simulink model "H250_LOEUnknown_400HzV3"  (R2022a)
settings: Solver=ode4  StartTime=0.0  StopTime=80  FixedStep=Ts  RelTol=1e-3
InitFcn:
  | H250_LOEUnknown_400HzParam
undefined symbols (not defined in the file or in its folder): DiscIntNeverNeededParam, Ts
libraries: sharedtransform x3, dspnetwork x1, pixhawk_slib_misc_utils x1
settings Model: Creator=kcx06  LastModifiedBy=kcx06
settings SolverCC: AlgebraicLoopSolver=TrustRegion  PositivePriorityOrder=on  AutoInsertRateTranBlk=on
settings DataIOCC: SaveOutput=off  DSMLogging=off  SaveTime=off  ReturnWorkspaceOutputs=off
settings OptimizationCC: DefaultParameterBehavior=Inlined  EnhancedBackFolding=on  PassReuseOutputArgsAs=Individual arguments  ZeroExternalMemoryAtStartup=off  ZeroInternalMemoryAtStartup=off  MaxStackSize=64  OptimizeBlockOrder=speed  DifferentSizesBufferReuse=on  OptimizationCustomize=off  EfficientTunableParamExpr=on
settings DebuggingCC: ParameterTunabilityLossMsg=error  UnconnectedInputMsg=warning  UnconnectedOutputMsg=warning  UnconnectedLineMsg=warning  SFMachineParentedDataDiag=warning
settings HardwareCC: ProdBitPerPointer=32  ProdBitPerSizeT=32  ProdBitPerPtrDiffT=32  ProdLargestAtomicInteger=Long  ProdLargestAtomicFloat=Double  ProdWordSize=32  ProdHWDeviceType=ARM Compatible->ARM Cortex
settings SFSimCC: MATLABDynamicMemAlloc=off
settings RTWCC: SystemTargetFile=ert.tlc  HardwareBoard=Pixhawk PX4  TLCOptions="-aInlineSetEventsForThisBaseRateFcn=TLC_FALSE -aSuppressMultiTaskScheduler=TLC_FALSE  -aRateBasedStepFcn=0"  TemplateMakefile=ert_default_tmf  GenerateReport=on  CustomSource=px4_simulink_app_params.c  Toolchain=Pixhawk Toolchain  BuildConfiguration=Faster Runs  LaunchReport=on  DLArmComputeVersion=19.05
settings CodeAppCC: ForceParamTrailComments=on  IgnoreCustomStorageClasses=off  OperatorAnnotations=on  SimulinkDataObjDesc=on  SFDataObjDesc=on  InsertBlockDesc=on
settings ERTTargetCC: SupportComplex=off  SupportContinuousTime=on  InlinedParameterPlacement=NonHierarchical  ERTCustomFileTemplate=px4_codertarget_file_process.tlc

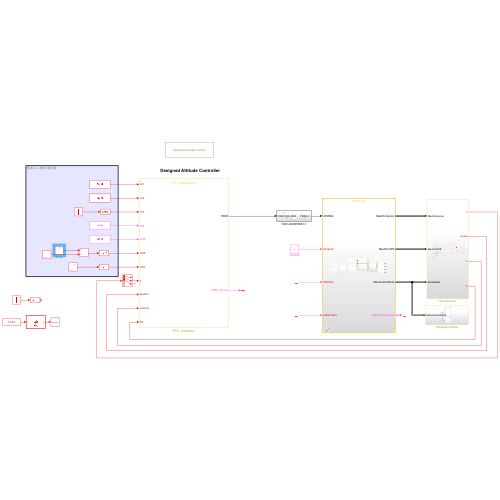
[thumbnail: Simulink's stored preview of the top-level diagram]
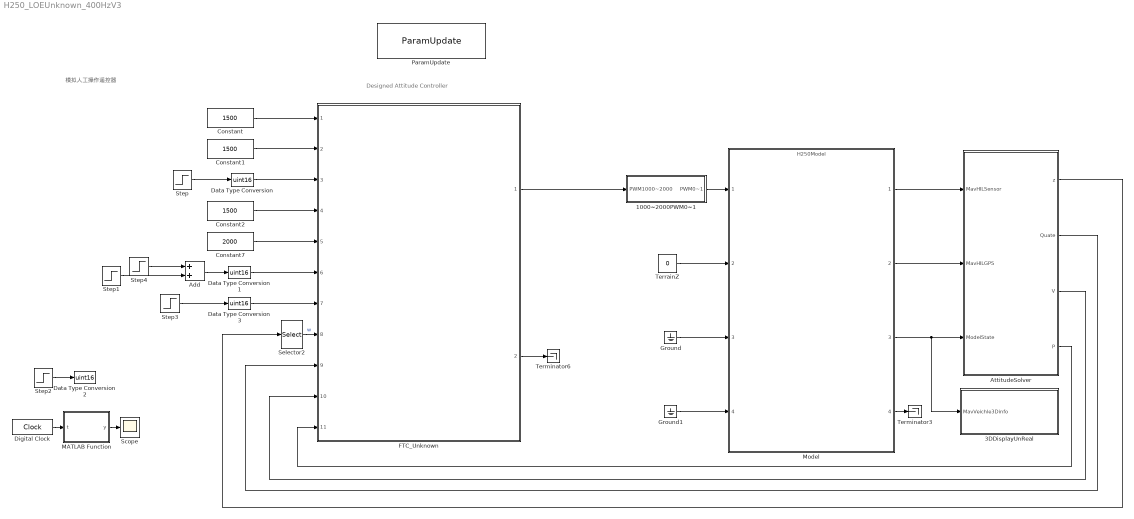
== system H250_LOEUnknown_400HzV3 ==
  note: Designed Attitude Controller
  note: 模拟人工操作遥控器
  1000~2000PWM0~1 : Subsystem
  3DDisplayUnReal : Subsystem
  Add : Sum
  AttitudeSolver : Subsystem
  Constant : Constant  Value=1500  OutDataTypeStr=uint16  SampleTime=Ts
  Constant1 : Constant  Value=1500  OutDataTypeStr=uint16  SampleTime=Ts
  Constant2 : Constant  Value=1500  OutDataTypeStr=uint16
  Constant7 : Constant  Value=2000  OutDataTypeStr=uint16
  Data Type Conversion{,1..3} (4 alike) : DataTypeConversion  OutDataTypeStr=uint16  SaturateOnIntegerOverflow=off  RndMeth=Floor
  Digital Clock : DigitalClock  SampleTime=Ts
  FTC_Unknown : Subsystem  SystemSampleTime=Ts  ReferencedSubsystem=FTC_UnknownV3
  Ground : Ground
  Ground1 : Ground
  MATLAB Function : MATLAB Function  TreatAsAtomicUnit=on
  Model : ModelReference  ModelNameDialog=H250Model.slx  SimulationMode=Normal  ModelReferenceVersion=5.4
  ParamUpdate : pixhawk_slib_misc_utils/ParamUpdate  Description=|  Unformatted_StrSet=0  TLC_StrSet=0  NumParams=0  Ts=0
      | ParamUpdate Block
      | 
      | Use this block at your top-level of your model to insert a "parameter update" function in the generated code.
      settings: SourceProductName=Pixhawk Target Blocks
  Scope : Scope
  Selector2 : Selector  IndexMode=Zero-based  InputPortWidth=6  IndexOptions=Index vector (dialog)  Indices=[0 1 2]  OutputSizes=1
  Step : Step  Time=15  Before=1900  After=1500  OutDataTypeStr=single  SampleTime=Ts
  Step1 : Step  Time=20  Before=1000  After=1500  OutDataTypeStr=single  SampleTime=Ts
  Step2 : Step  Time=20  Before=1500  After=1900  OutDataTypeStr=single  SampleTime=Ts
  Step3 : Step  Time=35  Before=1100  After=1500  OutDataTypeStr=single  SampleTime=Ts
  Step4 : Step  Time=20  After=500  OutDataTypeStr=single  SampleTime=Ts
  Terminator3 : Terminator
  Terminator6 : Terminator
  TerrainZ : Constant  Value=0
  wires:
  Model/1 -> AttitudeSolver/1(MavHILSensor)
  Ground/1 -> Model/3
  Model/2 -> AttitudeSolver/2(MavHILGPS)
  TerrainZ/1 -> Model/2
  Ground1/1 -> Model/4
  Model/4 -> Terminator3/1
  Model/3 -> AttitudeSolver/3(ModelState), 3DDisplayUnReal/1(MavVeichle3Dinfo)
  1000~2000PWM0~1/1(PWM0~1) -> Model/1
  FTC_Unknown/2 -> Terminator6/1
  Data Type Conversion1/1 -> FTC_Unknown/6
  Data Type Conversion/1 -> FTC_Unknown/3
  Constant2/1 -> FTC_Unknown/4
  Constant7/1 -> FTC_Unknown/5
  MATLAB Function/1(y) -> Scope/1
  Step/1 -> Data Type Conversion/1
  Constant/1 -> FTC_Unknown/1
  Digital Clock/1 -> MATLAB Function/1(t)
  Constant1/1 -> FTC_Unknown/2
  Selector2/1 -> FTC_Unknown/8  "w"
  Step1/1 -> Add/2
  FTC_Unknown/1 -> 1000~2000PWM0~1/1(PWM1000~2000)
  AttitudeSolver/4(P) -> FTC_Unknown/11
  AttitudeSolver/3(V) -> FTC_Unknown/10
  AttitudeSolver/2(Quate) -> FTC_Unknown/9
  AttitudeSolver/1(z) -> Selector2/1
  Step2/1 -> Data Type Conversion2/1
  Step3/1 -> Data Type Conversion3/1
  Data Type Conversion3/1 -> FTC_Unknown/7
  Step4/1 -> Add/1
  Add/1 -> Data Type Conversion1/1

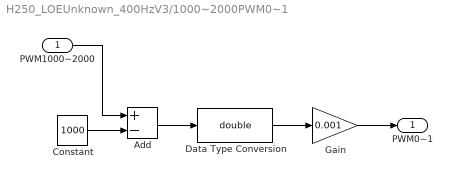
== system H250_LOEUnknown_400HzV3/1000~2000PWM0~1 ==
  PWM1000~2000 : Inport
  Add : Sum  Inputs=+-
  Constant : Constant  Value=1000
  Data Type Conversion : DataTypeConversion  OutDataTypeStr=double  SaturateOnIntegerOverflow=off  RndMeth=Floor
  Gain : Gain  Gain=0.001
  PWM0~1 : Outport
  wires:
  PWM1000~2000/1 -> Add/1
  Constant/1 -> Add/2
  Gain/1 -> PWM0~1/1
  Data Type Conversion/1 -> Gain/1
  Add/1 -> Data Type Conversion/1

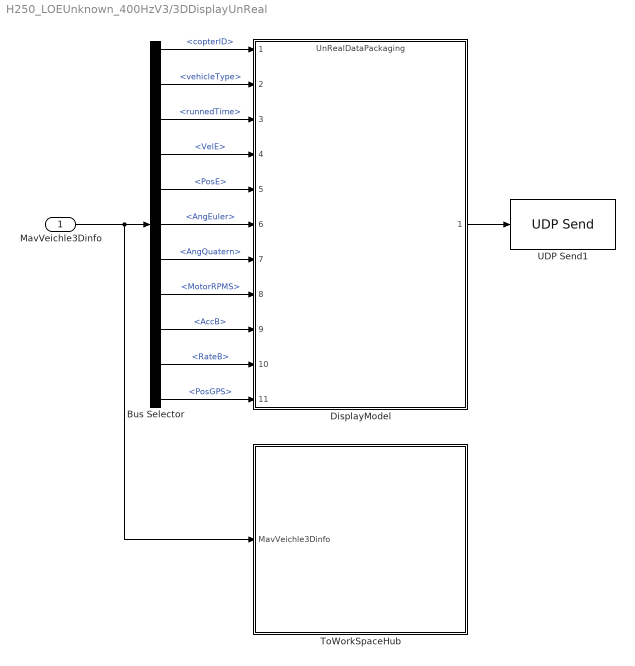
== system H250_LOEUnknown_400HzV3/3DDisplayUnReal ==
  MavVeichle3Dinfo : Inport
  Bus Selector : BusSelector  OutputSignals=copterID,vehicleType,runnedTime,VelE,PosE,AngEuler,AngQuatern,MotorRPMS,AccB,RateB,PosGPS
  DisplayModel : ModelReference  ModelNameDialog=UnRealDataPackaging.slx  ModelReferenceVersion=1.123
  ToWorkSpaceHub : Subsystem
  UDP Send1 : dspnetwork/UDP Send  remoteURL='127.0.0.1'  remotePort=20010  localURL='0.0.0.0'  localPortSource=Automatically determine  localPort=20011  sendBufferSize=8192  sampletime=-1  blockPlatform=[]  separateLengthPort=0
  wires:
  Bus Selector/10 -> DisplayModel/10  "<RateB>"
  Bus Selector/2 -> DisplayModel/2  "<vehicleType>"
  MavVeichle3Dinfo/1 -> ToWorkSpaceHub/1(MavVeichle3Dinfo), Bus Selector/1
  Bus Selector/8 -> DisplayModel/8  "<MotorRPMS>"
  Bus Selector/7 -> DisplayModel/7  "<AngQuatern>"
  Bus Selector/1 -> DisplayModel/1  "<copterID>"
  Bus Selector/6 -> DisplayModel/6  "<AngEuler>"
  Bus Selector/9 -> DisplayModel/9  "<AccB>"
  Bus Selector/5 -> DisplayModel/5  "<PosE>"
  Bus Selector/11 -> DisplayModel/11  "<PosGPS>"
  Bus Selector/3 -> DisplayModel/3  "<runnedTime>"
  Bus Selector/4 -> DisplayModel/4  "<VelE>"
  DisplayModel/1 -> UDP Send1/1

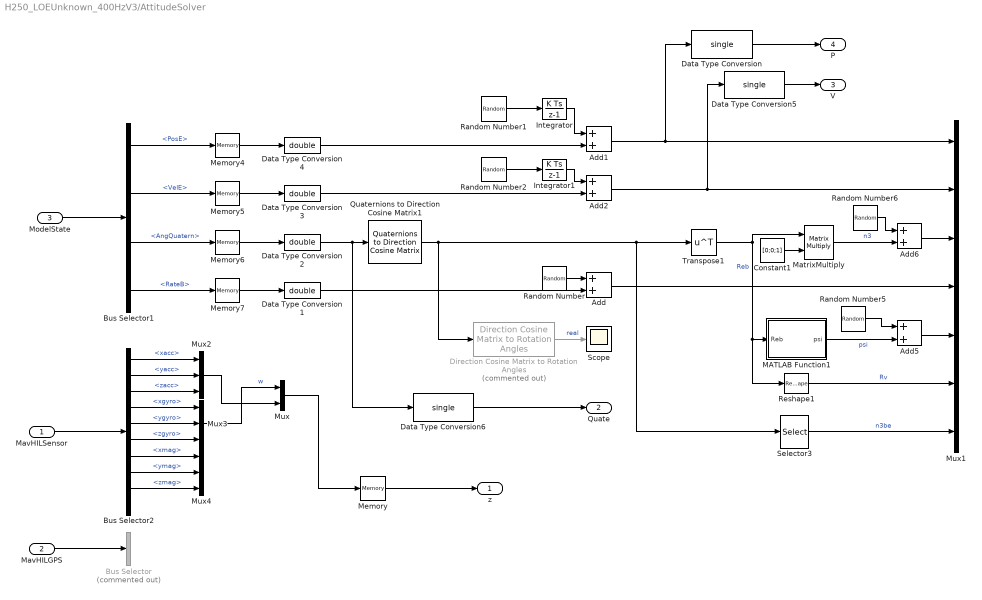
== system H250_LOEUnknown_400HzV3/AttitudeSolver ==
  MavHILSensor : Inport
  MavHILGPS : Inport  Port=2
  ModelState : Inport  Port=3
  Add{,1..2,5..6} (5 alike) : Sum
  Bus Selector : BusSelector  Commented=on  OutputSignals=lat,lon,alt,vn,ve,vd  OutputAsBus=on
  Bus Selector1 : BusSelector  OutputSignals=PosE,VelE,AngQuatern,RateB
  Bus Selector2 : BusSelector  OutputSignals=xacc,yacc,zacc,xgyro,ygyro,zgyro,xmag,ymag,zmag,pressure_alt
  Constant1 : Constant  Value=[0;0;1]
  Data Type Conversion : DataTypeConversion  OutDataTypeStr=single  SaturateOnIntegerOverflow=off  RndMeth=Floor
  Data Type Conversion{1..4} (4 alike) : DataTypeConversion  OutDataTypeStr=double  SaturateOnIntegerOverflow=off  RndMeth=Floor
  Data Type Conversion5 : DataTypeConversion  OutDataTypeStr=single  SaturateOnIntegerOverflow=off  RndMeth=Floor
  Data Type Conversion6 : DataTypeConversion  OutDataTypeStr=single  SaturateOnIntegerOverflow=off  RndMeth=Floor
  Direction Cosine Matrix to Rotation Angles : sharedtransform/Direction Cosine Matrix to Rotation Angles  Commented=on  rotationOrder=ZYX  aMode=aMode  action=None  tolerance=eps(2)
      settings: SourceProductBaseCode=AE,PW,DR,MT,VE
  Integrator : DiscreteIntegrator  SampleTime=Ts  ICPrevOutput=DiscIntNeverNeededParam  ICPrevScaledInput=DiscIntNeverNeededParam  mask(DiscretizedDiscreteIntegrator){}
      mask init:
      | %zoh
  Integrator1 : DiscreteIntegrator  SampleTime=Ts  ICPrevOutput=DiscIntNeverNeededParam  ICPrevScaledInput=DiscIntNeverNeededParam  mask(DiscretizedDiscreteIntegrator){}
      mask init:
      | %zoh
  MATLAB Function1 : MATLAB Function  TreatAsAtomicUnit=on
  MatrixMultiply : Product  Multiplication=Matrix(*)
  Memory : Memory
  Memory4 : Memory  InitialCondition=[0;0;0]
  Memory5 : Memory  InitialCondition=[0;0;0]
  Memory6 : Memory  InitialCondition=[1; 0; 0; 0]
  Memory7 : Memory  InitialCondition=[0;0;0]
  Mux : Mux  Inputs=2
  Mux1 : Mux  Inputs=[3 3 3 3 1 9 3]
  Mux2 : Mux  Inputs=3
  Mux3 : Mux  Inputs=3
  Mux4 : Mux  Inputs=3
  Quaternions to Direction Cosine Matrix1 : sharedtransform/Quaternions to  Direction Cosine Matrix  aMode=aMode
      settings: SourceProductBaseCode=AE,PW,DR,MT,VE
  Random Number : RandomNumber  Variance=0.001  Seed=[123 321 564]  SampleTime=Ts
  Random Number1 : RandomNumber  Variance=0.1  Seed=[10 20 15]  SampleTime=Ts
  Random Number2 : RandomNumber  Variance=0.1  Seed=[25 30 35]  SampleTime=Ts
  Random Number5 : RandomNumber  Variance=0.00002  Seed=[12]  SampleTime=Ts*4
  Random Number6 : RandomNumber  Variance=0.00002  Seed=[98 99 100]  SampleTime=Ts*4
  Reshape1 : Reshape
  Scope : Scope
  Selector3 : Selector  NumberOfDimensions=2  InputPortWidth=3  IndexOptions=Select all,Index vector (dialog)  Indices=[1 3],3  OutputSizes=1,1
  Transpose1 : Math  Operator=transpose
  z : Outport
  Quate : Outport  Port=2
  V : Outport  Port=3
  P : Outport  Port=4
  wires:
  Random Number/1 -> Add/1
  Integrator/1 -> Add1/1
  Random Number1/1 -> Integrator/1
  Random Number2/1 -> Integrator1/1
  Integrator1/1 -> Add2/1
  MavHILSensor/1 -> Bus Selector2/1
  Quaternions to Direction Cosine Matrix1/1 -> Direction Cosine Matrix to Rotation Angles/1, Selector3/1, Transpose1/1
  Bus Selector1/4 -> Memory7/1  "<RateB>"
  Add/1 -> Mux1/4
  Add2/1 -> Mux1/2, Data Type Conversion5/1
  Add1/1 -> Mux1/1, Data Type Conversion/1
  Add6/1 -> Mux1/3
  Transpose1/1 -> MatrixMultiply/1, MATLAB Function1/1(Reb), Reshape1/1  "Reb"
  Add5/1 -> Mux1/5
  Reshape1/1 -> Mux1/6  "Rv"
  MATLAB Function1/1(psi) -> Add5/2  "psi"
  MatrixMultiply/1 -> Add6/2  "n3"
  Random Number5/1 -> Add5/1
  Random Number6/1 -> Add6/1
  Selector3/1 -> Mux1/7  "n3be"
  Direction Cosine Matrix to Rotation Angles/1 -> Scope/1  "real"
  ModelState/1 -> Bus Selector1/1
  Bus Selector1/1 -> Memory4/1  "<PosE>"
  Bus Selector1/2 -> Memory5/1  "<VelE>"
  Bus Selector1/3 -> Memory6/1  "<AngQuatern>"
  MavHILGPS/1 -> Bus Selector/1
  Bus Selector2/1 -> Mux2/1  "<xacc>"
  Bus Selector2/2 -> Mux2/2  "<yacc>"
  Bus Selector2/3 -> Mux2/3  "<zacc>"
  Bus Selector2/5 -> Mux3/2  "<ygyro>"
  Bus Selector2/6 -> Mux3/3  "<zgyro>"
  Bus Selector2/4 -> Mux3/1  "<xgyro>"
  Bus Selector2/9 -> Mux4/3  "<zmag>"
  Bus Selector2/8 -> Mux4/2  "<ymag>"
  Bus Selector2/7 -> Mux4/1  "<xmag>"
  Data Type Conversion1/1 -> Add/2
  Data Type Conversion3/1 -> Add2/2
  Data Type Conversion4/1 -> Add1/2
  Memory4/1 -> Data Type Conversion4/1
  Memory5/1 -> Data Type Conversion3/1
  Memory6/1 -> Data Type Conversion2/1
  Memory7/1 -> Data Type Conversion1/1
  Constant1/1 -> MatrixMultiply/2
  Mux3/1 -> Mux/1  "w"
  Mux2/1 -> Mux/2
  Mux/1 -> Memory/1
  Data Type Conversion2/1 -> Data Type Conversion6/1, Quaternions to Direction Cosine Matrix1/1
  Data Type Conversion/1 -> P/1
  Data Type Conversion5/1 -> V/1
  Data Type Conversion6/1 -> Quate/1
  Memory/1 -> z/1

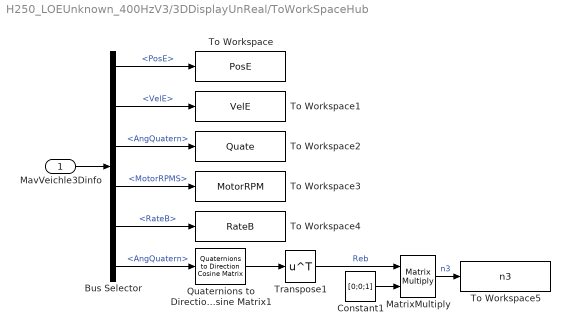
== system H250_LOEUnknown_400HzV3/3DDisplayUnReal/ToWorkSpaceHub ==
  MavVeichle3Dinfo : Inport
  Bus Selector : BusSelector  OutputSignals=PosE,VelE,AngQuatern,MotorRPMS,RateB,AngQuatern
  Constant1 : Constant  Value=[0;0;1]
  MatrixMultiply : Product  Multiplication=Matrix(*)
  Quaternions to Direction Cosine Matrix1 : sharedtransform/Quaternions to  Direction Cosine Matrix  aMode=aMode
      settings: SourceProductBaseCode=AE,PW,DR,MT,VE
  To Workspace : ToWorkspace  VariableName=PosE  SaveFormat=Timeseries  SampleTime=-1
  To Workspace1 : ToWorkspace  VariableName=VelE  SaveFormat=Timeseries  SampleTime=-1
  To Workspace2 : ToWorkspace  VariableName=Quate  SaveFormat=Timeseries  SampleTime=-1
  To Workspace3 : ToWorkspace  VariableName=MotorRPM  SaveFormat=Timeseries  SampleTime=-1
  To Workspace4 : ToWorkspace  VariableName=RateB  SaveFormat=Timeseries  SampleTime=-1
  To Workspace5 : ToWorkspace  VariableName=n3  SaveFormat=Timeseries  SampleTime=-1
  Transpose1 : Math  Operator=transpose
  wires:
  MavVeichle3Dinfo/1 -> Bus Selector/1
  Bus Selector/1 -> To Workspace/1  "<PosE>"
  Bus Selector/2 -> To Workspace1/1  "<VelE>"
  Bus Selector/3 -> To Workspace2/1  "<AngQuatern>"
  Bus Selector/4 -> To Workspace3/1  "<MotorRPMS>"
  Bus Selector/5 -> To Workspace4/1  "<RateB>"
  Constant1/1 -> MatrixMultiply/2
  Quaternions to Direction Cosine Matrix1/1 -> Transpose1/1
  Bus Selector/6 -> Quaternions to Direction Cosine Matrix1/1  "<AngQuatern>"
  Transpose1/1 -> MatrixMultiply/1  "Reb"
  MatrixMultiply/1 -> To Workspace5/1  "n3"

== matlab function H250_LOEUnknown_400HzV3/AttitudeSolver/MATLAB Function1 ==
  data: Reb input; psi output
function psi = fcn(Reb)
psi = atan2(Reb(2,1), Reb(1,1));

== matlab function H250_LOEUnknown_400HzV3/MATLAB Function ==
  data: y output; t input
function y = fcn(t)
y = 1000;

if t>=20
    y= 1400;
end

if t>=40
    y= 1600;
end

if t>=60
    y= 1800;
end

if t>=80
    y= 1800;
end
